simulink model "TCS_autosar"  (R2019b)
settings: Solver=VariableStepAuto  StartTime=0.0  StopTime=10.0  RelTol=1e-3
libraries: simulink x20
settings Model: Creator=12045  LastModifiedBy=12045
settings OptimizationCC: DefaultParameterBehavior=Inlined  EnhancedBackFolding=on  PassReuseOutputArgsAs=Individual arguments  ZeroExternalMemoryAtStartup=off  ZeroInternalMemoryAtStartup=off  OptimizeBlockOrder=speed  DifferentSizesBufferReuse=on  OptimizationCustomize=off  EfficientTunableParamExpr=on
settings DebuggingCC: ParameterTunabilityLossMsg=error
settings SFSimCC: SimGenImportedTypeDefs=on  MATLABDynamicMemAlloc=off
settings RTWCC: Description=AUTOSAR  SystemTargetFile=autosar.tlc  GenCodeOnly=on  TemplateMakefile=ert_default_tmf  GenerateReport=on  Toolchain=AUTOSAR Adaptive | CMake  IncludeHyperlinkInReport=on  LaunchReport=on  GenerateTraceInfo=on  GenerateTraceReport=on  GenerateTraceReportSl=on  GenerateTraceReportSf=on  GenerateTraceReportEml=on
settings CodeAppCC: ForceParamTrailComments=on  IgnoreCustomStorageClasses=off  MaxIdLength=63  OperatorAnnotations=on  SimulinkDataObjDesc=on  SFDataObjDesc=on  InsertBlockDesc=on
settings STFCustomTargetCC: TargetLangStandard=C99 (ISO)  MultiwordLength=256  ParMdlRefBuildCompliant=on  CompOptLevelCompliant=on  IncludeMdlTerminateFcn=off  CombineOutputUpdateFcns=on  SuppressErrorStatus=on  ERTCustomFileBanners=on  SupportNonFinite=off  SupportComplex=off  SupportContinuousTime=off  SupportNonInlinedSFcns=off  RemoveResetFunc=on  MATLABClassNameForMDSCustomization=Simulink.SoftwareTarget.ERTCustomization  AutosarCompliant=on  UseToolchainInfoCompliant=on  LookupTableObjectStructAxisOrder=2,1,3,4,...  LUTObjectStructOrderEvenSpacing=Size,Table,Breakpoints  SystemTargetFile=autosar.tlc
settings ERTTargetCC: TargetLangStandard=C99 (ISO)  ConcurrentExecutionCompliant=off  IncludeMdlTerminateFcn=off  SuppressErrorStatus=on  SupportNonFinite=off  SupportComplex=off  ModelStepFunctionPrototypeControlCompliant=off  CPPClassGenCompliant=off  AutosarCompliant=on  LookupTableObjectStructAxisOrder=2,1,3,4,...  LUTObjectStructOrderEvenSpacing=Size,Table,Breakpoints  InlinedParameterPlacement=NonHierarchical  ERTCustomFileTemplate=example_file_process.tlc

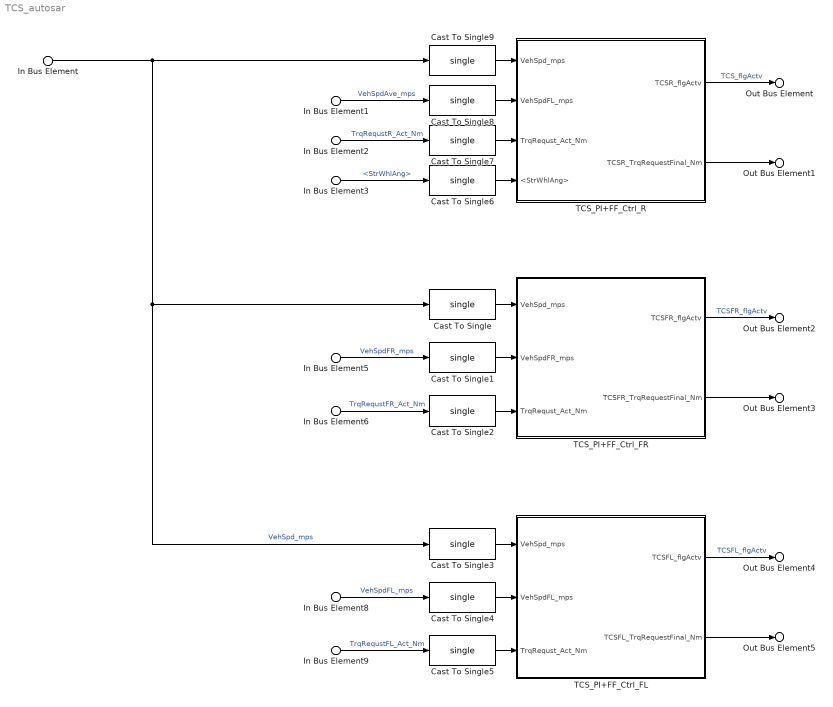
== system TCS_autosar ==
  In Bus Element : Inport  PortName=VehSpd_mps  Element=VehSpd_mps
  In Bus Element1 : Inport  Port=2  PortName=VehSpdAve_mps  Element=VehSpdAve_mps
  In Bus Element2 : Inport  Port=3  PortName=TrqRequstR_Act_Nm  Element=TrqRequstR_Act_Nm
  In Bus Element3 : Inport  Port=4  PortName=StrWhlAng  Element=StrWhlAng
  In Bus Element5 : Inport  Port=5  PortName=VehSpdFR_mps  Element=VehSpdFR_mps
  In Bus Element6 : Inport  Port=6  PortName=TrqRequstFR_Act_Nm  Element=TrqRequstFR_Act_Nm
  In Bus Element8 : Inport  Port=7  PortName=VehSpdFL_mps1  Element=VehSpdFL_mpsVehSpdFL_mps1
  In Bus Element9 : Inport  Port=8  PortName=TrqRequst_Act_Nm2  Element=TrqRequstFL_Act_NmTrqRequstFL_Act_Nm
  Cast To Single{,1..9} (10 alike) : DataTypeConversion  OutDataTypeStr=single
  TCS_PI+FF_Ctrl_FL : Subsystem
  TCS_PI+FF_Ctrl_FR : Subsystem
  TCS_PI+FF_Ctrl_R : Subsystem
  Out Bus Element : Outport  PortName=TCS_flgActv_R  Element=TCS_flgActv_R
  Out Bus Element1 : Outport  Port=2  PortName=TCSR_TrqRequestFinal_Nm  Element=TCSR_TrqRequestFinal_Nm
  Out Bus Element2 : Outport  Port=3  PortName=TCS_flgActv_FR  Element=TCS_flgActv_FR
  Out Bus Element3 : Outport  Port=4  PortName=TCSFR_TrqRequestFinal_Nm  Element=TCSFR_TrqRequestFinal_Nm
  Out Bus Element4 : Outport  Port=5  PortName=TCS_flgActv_FL  Element=TCS_flgActv_FL
  Out Bus Element5 : Outport  Port=6  PortName=TCSFL_TrqRequestFinal_Nm  Element=TCSFL_TrqRequestFinal_Nm
  wires:
  Cast To Single/1 -> TCS_PI+FF_Ctrl_FR/1(VehSpd_mps)
  Cast To Single1/1 -> TCS_PI+FF_Ctrl_FR/2(VehSpdFR_mps)
  Cast To Single2/1 -> TCS_PI+FF_Ctrl_FR/3(TrqRequst_Act_Nm)
  Cast To Single3/1 -> TCS_PI+FF_Ctrl_FL/1(VehSpd_mps)
  Cast To Single4/1 -> TCS_PI+FF_Ctrl_FL/2(VehSpdFL_mps)
  Cast To Single5/1 -> TCS_PI+FF_Ctrl_FL/3(TrqRequst_Act_Nm)
  Cast To Single6/1 -> TCS_PI+FF_Ctrl_R/4(<StrWhlAng>)
  Cast To Single7/1 -> TCS_PI+FF_Ctrl_R/3(TrqRequst_Act_Nm)
  Cast To Single8/1 -> TCS_PI+FF_Ctrl_R/2(VehSpdFL_mps)
  Cast To Single9/1 -> TCS_PI+FF_Ctrl_R/1(VehSpd_mps)
  In Bus Element/1 -> Cast To Single3/1, Cast To Single/1, Cast To Single9/1  "VehSpd_mps"
  In Bus Element1/1 -> Cast To Single8/1  "VehSpdAve_mps"
  In Bus Element2/1 -> Cast To Single7/1  "TrqRequstR_Act_Nm"
  In Bus Element3/1 -> Cast To Single6/1  "<StrWhlAng>"
  In Bus Element5/1 -> Cast To Single1/1  "VehSpdFR_mps"
  In Bus Element6/1 -> Cast To Single2/1  "TrqRequstFR_Act_Nm"
  In Bus Element8/1 -> Cast To Single4/1  "VehSpdFL_mps"
  In Bus Element9/1 -> Cast To Single5/1  "TrqRequstFL_Act_Nm"
  TCS_PI+FF_Ctrl_R/1(TCSR_flgActv) -> Out Bus Element/1  "TCS_flgActv"
  TCS_PI+FF_Ctrl_R/2(TCSR_TrqRequestFinal_Nm) -> Out Bus Element1/1
  TCS_PI+FF_Ctrl_FR/1(TCSFR_flgActv) -> Out Bus Element2/1  "TCSFR_flgActv"
  TCS_PI+FF_Ctrl_FR/2(TCSFR_TrqRequestFinal_Nm) -> Out Bus Element3/1
  TCS_PI+FF_Ctrl_FL/1(TCSFL_flgActv) -> Out Bus Element4/1  "TCSFL_flgActv"
  TCS_PI+FF_Ctrl_FL/2(TCSFL_TrqRequestFinal_Nm) -> Out Bus Element5/1

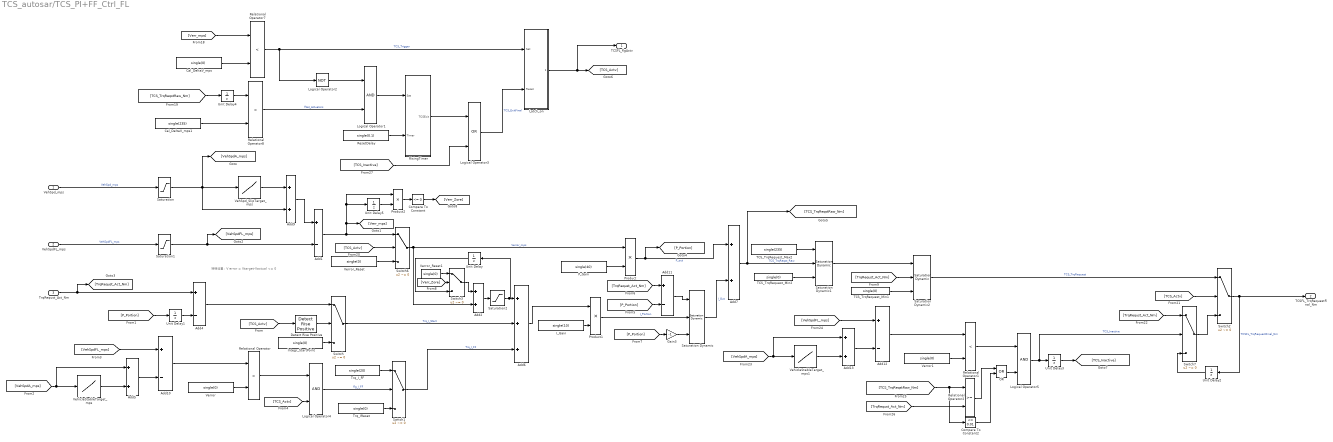
== system TCS_autosar/TCS_PI+FF_Ctrl_FL ==
  note: 特殊设置：V error = Vtarget-Vactual <= 0
  VehSpd_mps : Inport
  VehSpdFL_mps : Inport  Port=2
  TrqRequst_Act_Nm : Inport  Port=3
  Add{1,4,10..12} (5 alike) : Sum  Inputs=+-
  Add{2,5,7,9,13} (5 alike) : Sum
  Add6 : Sum  Inputs=+++
  Cal_DeltaV_mps : Constant  Value=single(0)
  Cal_DeltaV_mps1 : Constant  Value=single(235)
  Compare To Constant : simulink/Logic and Bit Operations/Compare To Constant  relop=<=  const=0  OutDataTypeStr=boolean
  Compare To Constant2 : simulink/Logic and Bit Operations/Compare To Constant  relop=<=  const=0.01  OutDataTypeStr=boolean
  Detect Rise Positive : simulink/Logic and Bit Operations/Detect Rise Positive  vinit=0  OutDataTypeStr=boolean
  Gain3 : Gain  Gain=-1
  I_Gain : Constant  Value=single(10)
  Integr_StartPoint : Constant  Value=single(0)
  Latch_on : Subsystem
  Logical Operator1 : Logic  AllPortsSameDT=off  OutDataTypeStr=boolean
  Logical Operator2 : Logic  Operator=NOT  AllPortsSameDT=off  OutDataTypeStr=boolean
  Logical Operator3 : Logic  Operator=OR  AllPortsSameDT=off  OutDataTypeStr=boolean
  Logical Operator4 : Logic  AllPortsSameDT=off  OutDataTypeStr=boolean
  Logical Operator5 : Logic  AllPortsSameDT=off  OutDataTypeStr=boolean
  OR : Logic  Operator=OR  AllPortsSameDT=off  OutDataTypeStr=boolean
  P_Gain : Constant  Value=single(40)
  Product : Product
  Product1 : Product
  Product2 : Product
  Relational Operator : RelationalOperator  Operator=<  OutDataTypeStr=boolean  RndMeth=Simplest
  Relational Operator1 : RelationalOperator  Operator=<  OutDataTypeStr=boolean  RndMeth=Simplest
  Relational Operator2 : RelationalOperator  OutDataTypeStr=boolean  RndMeth=Simplest
  Relational Operator7 : RelationalOperator  Operator=<  OutDataTypeStr=boolean  RndMeth=Simplest
  Relational Operator8 : RelationalOperator  Operator=>  OutDataTypeStr=boolean  RndMeth=Simplest
  ResetDelay : Constant  Value=single(0.1)
  RisingTimer : Subsystem
  Saturation : Saturate  UpperLimit=40  LowerLimit=0
  Saturation Dynamic : simulink/Discontinuities/Saturation Dynamic  OutMin=[]  OutMax=[]  OutDataTypeStr=Inherit: Same as second input  OutDataType=fixdt(1, 16)  OutScaling=2^-10  DoSatur=off
  Saturation Dynamic1 : simulink/Discontinuities/Saturation Dynamic  OutMin=[]  OutMax=[]  OutDataTypeStr=Inherit: Same as second input  OutDataType=fixdt(1, 16)  OutScaling=2^-10  DoSatur=off
  Saturation Dynamic2 : simulink/Discontinuities/Saturation Dynamic  OutMin=[]  OutMax=[]  OutDataTypeStr=Inherit: Same as second input  OutDataType=fixdt(1, 16)  OutScaling=2^-10  DoSatur=off
  Saturation1 : Saturate  UpperLimit=50  LowerLimit=0
  Saturation2 : Saturate  UpperLimit=400  LowerLimit=-100
  Switch{,1..3,6..7} (6 alike) : Switch  Criteria=u2 ~= 0
  TCS_TrqRequest_Max2 : Constant  Value=single(235)
  TCS_TrqRequest_Min1 : Constant  Value=single(0)
  TCS_TrqRequest_Min2 : Constant  Value=single(0)
  Trq_IReset : Constant  Value=single(0)
  Trq_I_FF : Constant  Value=single(20)
  Unit Delay{,1..5} (6 alike) : UnitDelay  SampleTime=-1  HasFrameUpgradeWarning=on
  VehSpd_SlipTarget_mps : Lookup_n-D  NumberOfTableDimensions=1  BreakpointsForDimension1=[0,3,25,30]  Table=[0.3,0.3,2.5,2.5]  ExtrapMethod=Clip  InternalRulePriority=Speed  RndMeth=Simplest  InputSameDT=on
  VehicleStableTarget_mps : Lookup_n-D  NumberOfTableDimensions=1  BreakpointsForDimension1=[0,3,25,30]  Table=[0.4,0.4,1.2,1.2]  ExtrapMethod=Clip  InternalRulePriority=Speed  RndMeth=Simplest  InputSameDT=on
  VehicleStableTarget_mps1 : Lookup_n-D  NumberOfTableDimensions=1  BreakpointsForDimension1=[0,3,25,30]  Table=[0.4,0.4,1.2,1.2]  ExtrapMethod=Clip  InternalRulePriority=Speed  RndMeth=Simplest  InputSameDT=on
  Verror : Constant  Value=single(0)
  Verror1 : Constant  Value=single(0)
  Verror_Reset : Constant  Value=single(0)
  Verror_Reset1 : Constant  Value=single(0)
  TCSFL_flgActv : Outport
  TCSFL_TrqRequestFinal_Nm : Outport  Port=2
  wires:
  Switch2/1 -> TCSFL_TrqRequestFinal_Nm/1, Unit Delay2/1  "TCSFL_TrqRequestFinal_Nm"
  Saturation/1 -> Add9/2, VehSpd_SlipTarget_mps/1, [VehSpdA_mps]
  Gain3/1 -> Saturation Dynamic/3
  [P_Portion] -> Gain3/1
  P_Gain/1 -> Product/2
  Unit Delay/1 -> Switch3/3
  Add2/1 -> Saturation2/1
  [TrqRequst_Act_Nm] -> Add11/1
  Saturation2/1 -> Unit Delay/1, Add6/1
  Switch/1 -> Add6/2  "Trq_I_Start"
  Saturation Dynamic/1 -> Add7/2  "I_Out"
  VehSpd_mps/1 -> Saturation/1  "VehSpd_mps"
  Saturation1/1 -> Add1/2, [VehSpdFL_mps]
  Product1/1 -> Saturation Dynamic/2  "I_Portion"
  TrqRequst_Act_Nm/1 -> Add4/1, [TrqRequst_Act_Nm]
  Add6/1 -> Product1/1
  TCS_TrqRequest_Min1/1 -> Saturation Dynamic2/3
  Detect Rise Positive/1 -> Switch/2
  Integr_StartPoint/1 -> Switch/3
  I_Gain/1 -> Product1/2
  Saturation Dynamic2/1 -> Switch2/1  "TCS_TrqRequest"
  Add7/1 -> Saturation Dynamic1/2, [TCS_TrqReqstRaw_Nm]  "TCS_TrqReqst_Raw"
  [TrqRequst_Act_Nm] -> Saturation Dynamic2/2
  VehSpd_SlipTarget_mps/1 -> Add9/1
  Add9/1 -> Add1/1
  [Verr_mps] -> Relational Operator7/1
  Cal_DeltaV_mps/1 -> Relational Operator7/2
  Relational Operator7/1 -> Latch_on/1(Set), Logical Operator2/1  "TCS_Trigger"
  [TCS_TrqReqstRaw_Nm] -> Unit Delay4/1
  Logical Operator2/1 -> Logical Operator1/1
  Relational Operator8/1 -> Logical Operator1/2  "fSat_Actuators"
  Cal_DeltaV_mps1/1 -> Relational Operator8/2
  Logical Operator1/1 -> RisingTimer/1(Set)
  ResetDelay/1 -> RisingTimer/2(Timer)
  RisingTimer/1(TCSExit) -> Logical Operator3/1
  Logical Operator3/1 -> Latch_on/2(Reset)  "TCS_ExitFinal"
  Latch_on/1(flg_TCSActv) -> TCSFL_flgActv/1, [TCS_Actv]
  [TCS_Actv] -> Switch6/2
  Verror_Reset/1 -> Switch6/3
  Switch6/1 -> Product/1, Add2/2  "Verror_mps"
  Product/1 -> [P_Portion], Add7/1  "P_out"
  [TCS_Actv] -> Detect Rise Positive/1
  [P_Portion] -> Unit Delay1/1
  Add4/1 -> Switch/1
  Unit Delay1/1 -> Add4/2
  [VehSpdA_mps] -> Add5/1, VehicleStableTarget_mps/1
  VehicleStableTarget_mps/1 -> Add5/2
  Add5/1 -> Add10/2
  [VehSpdFL_mps] -> Add10/1
  Add10/1 -> Relational Operator/1
  Verror/1 -> Relational Operator/2
  Relational Operator/1 -> Logical Operator4/1
  [TCS_Actv] -> Logical Operator4/2
  Logical Operator4/1 -> Switch1/2  "flg_I_FF"
  Trq_I_FF/1 -> Switch1/1
  Trq_IReset/1 -> Switch1/3
  Switch1/1 -> Add6/3  "Trq_I_FF"
  [P_Portion] -> Add11/2
  Add11/1 -> Saturation Dynamic/1
  [TCS_Actv] -> Switch2/2
  Switch7/1 -> Switch2/3
  [TrqRequst_Act_Nm] -> Switch7/1
  Verror1/1 -> Relational Operator1/2
  Add12/1 -> Relational Operator1/1
  [VehSpdFL_mps] -> Add12/1
  Add13/1 -> Add12/2
  VehicleStableTarget_mps1/1 -> Add13/2
  [VehSpdA_mps] -> VehicleStableTarget_mps1/1, Add13/1
  [TCS_TrqReqstRaw_Nm] -> Compare To Constant2/1, Relational Operator2/1
  [TrqRequst_Act_Nm] -> Relational Operator2/2
  Relational Operator1/1 -> Logical Operator5/1
  Logical Operator5/1 -> Switch7/2, Unit Delay3/1  "TCS_Inactive"
  Unit Delay3/1 -> [TCS_Inactive]
  [TCS_Inactive] -> Logical Operator3/2
  Unit Delay4/1 -> Relational Operator8/1
  VehSpdFL_mps/1 -> Saturation1/1  "VehSpdFL_mps"
  Saturation Dynamic1/1 -> Saturation Dynamic2/1
  TCS_TrqRequest_Max2/1 -> Saturation Dynamic1/1
  TCS_TrqRequest_Min2/1 -> Saturation Dynamic1/3
  Switch3/1 -> Add2/1
  Verror_Reset1/1 -> Switch3/1
  [Verr_Zore] -> Switch3/2
  Product2/1 -> Compare To Constant/1
  Unit Delay5/1 -> Product2/2
  Add1/1 -> Switch6/1, [Verr_mps], Unit Delay5/1, Product2/1
  Compare To Constant/1 -> [Verr_Zore]
  Unit Delay2/1 -> Switch7/3
  Compare To Constant2/1 -> OR/2
  Relational Operator2/1 -> OR/1
  OR/1 -> Logical Operator5/2

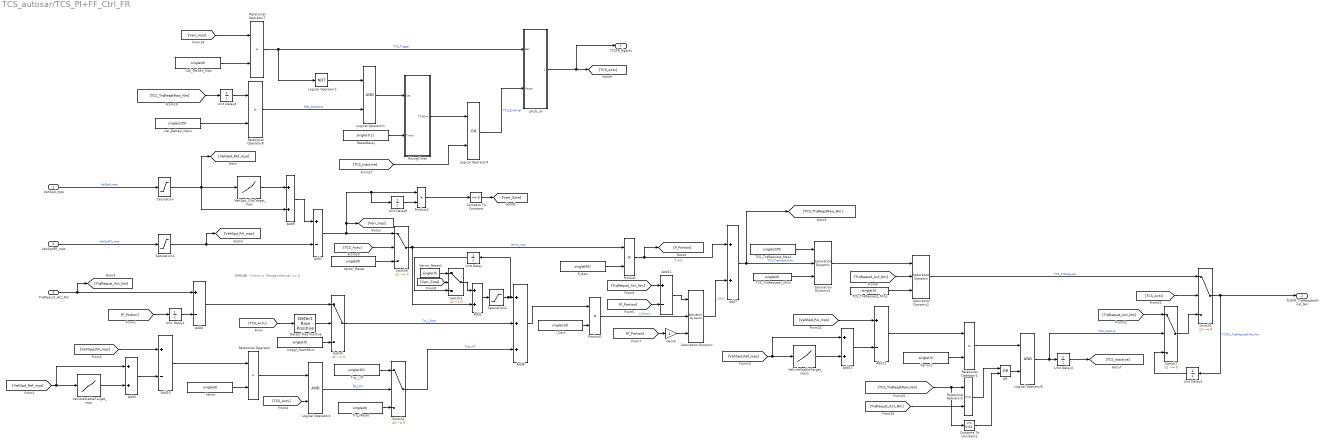
== system TCS_autosar/TCS_PI+FF_Ctrl_FR ==
  note: 特殊设置：V error = Vtarget-Vactual <= 0
  VehSpd_mps : Inport
  VehSpdFR_mps : Inport  Port=2
  TrqRequst_Act_Nm : Inport  Port=3
  Add{1,4,10..12} (5 alike) : Sum  Inputs=+-
  Add{2,5,7,9,13} (5 alike) : Sum
  Add6 : Sum  Inputs=+++
  Cal_DeltaV_mps : Constant  Value=single(0)
  Cal_DeltaV_mps1 : Constant  Value=single(235)
  Compare To Constant : simulink/Logic and Bit Operations/Compare To Constant  relop=<=  const=0  OutDataTypeStr=boolean
  Compare To Constant2 : simulink/Logic and Bit Operations/Compare To Constant  relop=<=  const=0.01  OutDataTypeStr=boolean
  Detect Rise Positive : simulink/Logic and Bit Operations/Detect Rise Positive  vinit=0  OutDataTypeStr=boolean
  Gain3 : Gain  Gain=-1
  I_Gain : Constant  Value=single(10)
  Integr_StartPoint : Constant  Value=single(0)
  Latch_on : Subsystem
  Logical Operator1 : Logic  AllPortsSameDT=off  OutDataTypeStr=boolean
  Logical Operator2 : Logic  Operator=NOT  AllPortsSameDT=off  OutDataTypeStr=boolean
  Logical Operator3 : Logic  Operator=OR  AllPortsSameDT=off  OutDataTypeStr=boolean
  Logical Operator4 : Logic  AllPortsSameDT=off  OutDataTypeStr=boolean
  Logical Operator5 : Logic  AllPortsSameDT=off  OutDataTypeStr=boolean
  OR : Logic  Operator=OR  AllPortsSameDT=off  OutDataTypeStr=boolean
  P_Gain : Constant  Value=single(40)
  Product : Product
  Product1 : Product
  Product2 : Product
  Relational Operator : RelationalOperator  Operator=<  OutDataTypeStr=boolean  RndMeth=Simplest
  Relational Operator1 : RelationalOperator  Operator=<  OutDataTypeStr=boolean  RndMeth=Simplest
  Relational Operator2 : RelationalOperator  OutDataTypeStr=boolean  RndMeth=Simplest
  Relational Operator7 : RelationalOperator  Operator=<  OutDataTypeStr=boolean  RndMeth=Simplest
  Relational Operator8 : RelationalOperator  Operator=>  OutDataTypeStr=boolean  RndMeth=Simplest
  ResetDelay : Constant  Value=single(0.1)
  RisingTimer : Subsystem
  Saturation : Saturate  UpperLimit=40  LowerLimit=0
  Saturation Dynamic : simulink/Discontinuities/Saturation Dynamic  OutMin=[]  OutMax=[]  OutDataTypeStr=Inherit: Same as second input  OutDataType=fixdt(1, 16)  OutScaling=2^-10  DoSatur=off
  Saturation Dynamic1 : simulink/Discontinuities/Saturation Dynamic  OutMin=[]  OutMax=[]  OutDataTypeStr=Inherit: Same as second input  OutDataType=fixdt(1, 16)  OutScaling=2^-10  DoSatur=off
  Saturation Dynamic2 : simulink/Discontinuities/Saturation Dynamic  OutMin=[]  OutMax=[]  OutDataTypeStr=Inherit: Same as second input  OutDataType=fixdt(1, 16)  OutScaling=2^-10  DoSatur=off
  Saturation1 : Saturate  UpperLimit=50  LowerLimit=0
  Saturation2 : Saturate  UpperLimit=400  LowerLimit=-100
  Switch{,1..3,6..7} (6 alike) : Switch  Criteria=u2 ~= 0
  TCS_TrqRequest_Max2 : Constant  Value=single(235)
  TCS_TrqRequest_Min1 : Constant  Value=single(0)
  TCS_TrqRequest_Min2 : Constant  Value=single(0)
  Trq_IReset : Constant  Value=single(0)
  Trq_I_FF : Constant  Value=single(20)
  Unit Delay{,1..5} (6 alike) : UnitDelay  SampleTime=-1  HasFrameUpgradeWarning=on
  VehSpd_SlipTarget_mps : Lookup_n-D  NumberOfTableDimensions=1  BreakpointsForDimension1=[0,3,25,30]  Table=[0.3,0.3,2.5,2.5]  ExtrapMethod=Clip  InternalRulePriority=Speed  RndMeth=Simplest  InputSameDT=on
  VehicleStableTarget_mps : Lookup_n-D  NumberOfTableDimensions=1  BreakpointsForDimension1=[0,3,25,30]  Table=[0.4,0.4,1.2,1.2]  ExtrapMethod=Clip  InternalRulePriority=Speed  RndMeth=Simplest  InputSameDT=on
  VehicleStableTarget_mps1 : Lookup_n-D  NumberOfTableDimensions=1  BreakpointsForDimension1=[0,3,25,30]  Table=[0.4,0.4,1.2,1.2]  ExtrapMethod=Clip  InternalRulePriority=Speed  RndMeth=Simplest  InputSameDT=on
  Verror : Constant  Value=single(0)
  Verror1 : Constant  Value=single(0)
  Verror_Reset : Constant  Value=single(0)
  Verror_Reset1 : Constant  Value=single(0)
  TCSFR_flgActv : Outport
  TCSFR_TrqRequestFinal_Nm : Outport  Port=2
  wires:
  [Verr_Zore] -> Switch3/2
  Verror_Reset1/1 -> Switch3/1
  Switch3/1 -> Add2/1
  TCS_TrqRequest_Min2/1 -> Saturation Dynamic1/3
  TCS_TrqRequest_Max2/1 -> Saturation Dynamic1/1
  Saturation Dynamic1/1 -> Saturation Dynamic2/1
  VehSpdFR_mps/1 -> Saturation1/1  "VehSpdFL_mps"
  Unit Delay4/1 -> Relational Operator8/1
  [TCS_Inactive] -> Logical Operator3/2
  Unit Delay3/1 -> [TCS_Inactive]
  Logical Operator5/1 -> Switch7/2, Unit Delay3/1  "TCS_Inactive"
  Relational Operator1/1 -> Logical Operator5/1
  [TrqRequst_Act_Nm] -> Relational Operator2/2
  [TCS_TrqReqstRaw_Nm] -> Compare To Constant2/1, Relational Operator2/1
  [VehSpd_Ref_mps] -> Add13/1, VehicleStableTarget_mps1/1
  VehicleStableTarget_mps1/1 -> Add13/2
  Add13/1 -> Add12/2
  [VehSpd_RA_mps] -> Add12/1
  Add12/1 -> Relational Operator1/1
  Verror1/1 -> Relational Operator1/2
  [TrqRequst_Act_Nm] -> Switch7/1
  Switch7/1 -> Switch2/3
  [TCS_Actv] -> Switch2/2
  Add11/1 -> Saturation Dynamic/1
  [P_Portion] -> Add11/2
  Switch1/1 -> Add6/3  "Trq_I_FF"
  Trq_IReset/1 -> Switch1/3
  Trq_I_FF/1 -> Switch1/1
  Logical Operator4/1 -> Switch1/2  "flg_I_FF"
  [TCS_Actv] -> Logical Operator4/2
  Relational Operator/1 -> Logical Operator4/1
  Verror/1 -> Relational Operator/2
  Add10/1 -> Relational Operator/1
  [VehSpd_RA_mps] -> Add10/1
  Add5/1 -> Add10/2
  VehicleStableTarget_mps/1 -> Add5/2
  [VehSpd_Ref_mps] -> VehicleStableTarget_mps/1, Add5/1
  Unit Delay1/1 -> Add4/2
  Add4/1 -> Switch/1
  [P_Portion] -> Unit Delay1/1
  [TCS_Actv] -> Detect Rise Positive/1
  Product/1 -> Add7/1, [P_Portion]  "P_out"
  Switch6/1 -> Add2/2, Product/1  "Verror_mps"
  Verror_Reset/1 -> Switch6/3
  [TCS_Actv] -> Switch6/2
  Latch_on/1(flg_TCSActv) -> [TCS_Actv], TCSFR_flgActv/1
  Logical Operator3/1 -> Latch_on/2(Reset)  "TCS_ExitFinal"
  RisingTimer/1(TCSExit) -> Logical Operator3/1
  ResetDelay/1 -> RisingTimer/2(Timer)
  Logical Operator1/1 -> RisingTimer/1(Set)
  Cal_DeltaV_mps1/1 -> Relational Operator8/2
  Relational Operator8/1 -> Logical Operator1/2  "fSat_Actuators"
  Logical Operator2/1 -> Logical Operator1/1
  [TCS_TrqReqstRaw_Nm] -> Unit Delay4/1
  Relational Operator7/1 -> Logical Operator2/1, Latch_on/1(Set)  "TCS_Trigger"
  Cal_DeltaV_mps/1 -> Relational Operator7/2
  [Verr_mps] -> Relational Operator7/1
  Add9/1 -> Add1/1
  VehSpd_SlipTarget_mps/1 -> Add9/1
  [TrqRequst_Act_Nm] -> Saturation Dynamic2/2
  Add7/1 -> [TCS_TrqReqstRaw_Nm], Saturation Dynamic1/2  "TCS_TrqReqst_Raw"
  Saturation Dynamic2/1 -> Switch2/1  "TCS_TrqRequest"
  I_Gain/1 -> Product1/2
  Integr_StartPoint/1 -> Switch/3
  Detect Rise Positive/1 -> Switch/2
  TCS_TrqRequest_Min1/1 -> Saturation Dynamic2/3
  Add6/1 -> Product1/1
  TrqRequst_Act_Nm/1 -> [TrqRequst_Act_Nm], Add4/1
  Product1/1 -> Saturation Dynamic/2  "I_Portion"
  Saturation1/1 -> [VehSpd_RA_mps], Add1/2
  VehSpd_mps/1 -> Saturation/1  "VehSpd_mps"
  Saturation Dynamic/1 -> Add7/2  "I_Out"
  Switch/1 -> Add6/2  "Trq_I_Start"
  Saturation2/1 -> Add6/1, Unit Delay/1
  [TrqRequst_Act_Nm] -> Add11/1
  Add2/1 -> Saturation2/1
  Unit Delay/1 -> Switch3/3
  P_Gain/1 -> Product/2
  [P_Portion] -> Gain3/1
  Gain3/1 -> Saturation Dynamic/3
  Saturation/1 -> [VehSpd_Ref_mps], VehSpd_SlipTarget_mps/1, Add9/2
  Switch2/1 -> Unit Delay2/1, TCSFR_TrqRequestFinal_Nm/1  "TCSFL_TrqRequestFinal_Nm"
  Product2/1 -> Compare To Constant/1
  Unit Delay5/1 -> Product2/2
  Add1/1 -> Unit Delay5/1, Product2/1, [Verr_mps], Switch6/1
  Compare To Constant/1 -> [Verr_Zore]
  Unit Delay2/1 -> Switch7/3
  Compare To Constant2/1 -> OR/2
  Relational Operator2/1 -> OR/1
  OR/1 -> Logical Operator5/2

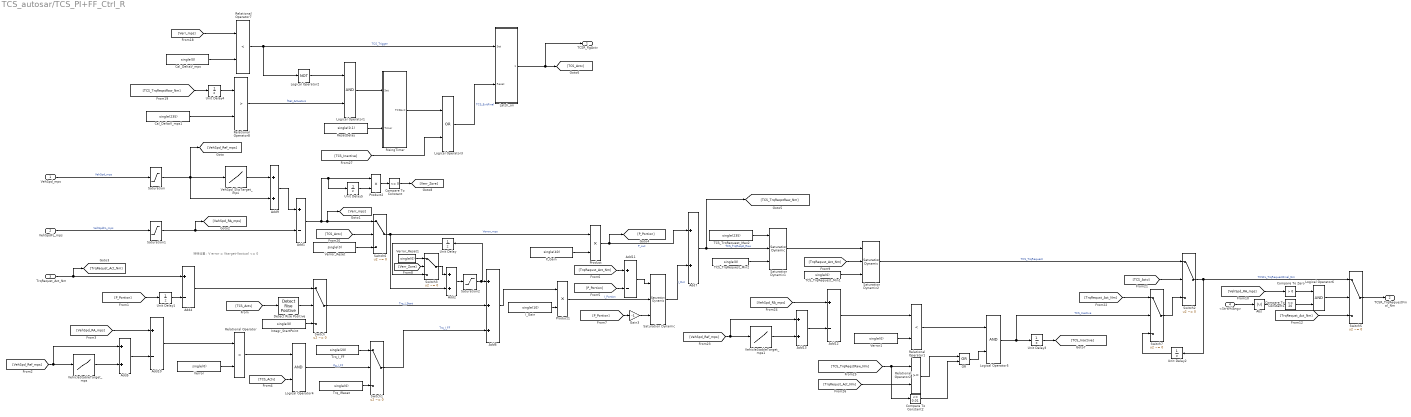
== system TCS_autosar/TCS_PI+FF_Ctrl_R ==
  note: 特殊设置：V error = Vtarget-Vactual <= 0
  VehSpd_mps : Inport
  VehSpdFL_mps : Inport  Port=2
  TrqRequst_Act_Nm : Inport  Port=3
  <StrWhlAng> : Inport  Port=4
  Abs : Abs
  Add{1,4,10..12} (5 alike) : Sum  Inputs=+-
  Add{2,5,7,9,13} (5 alike) : Sum
  Add6 : Sum  Inputs=+++
  Cal_DeltaV_mps : Constant  Value=single(0)
  Cal_DeltaV_mps1 : Constant  Value=single(235)
  Compare To Constant : simulink/Logic and Bit Operations/Compare To Constant  relop=<=  const=0  OutDataTypeStr=boolean
  Compare To Constant1 : simulink/Logic and Bit Operations/Compare To Constant  relop=<=  const=20  OutDataTypeStr=boolean
  Compare To Constant2 : simulink/Logic and Bit Operations/Compare To Constant  relop=<=  const=0.01  OutDataTypeStr=boolean
  Compare To Zero : simulink/Logic and Bit Operations/Compare To Zero  relop=>  OutDataTypeStr=boolean
  Detect Rise Positive : simulink/Logic and Bit Operations/Detect Rise Positive  vinit=0  OutDataTypeStr=boolean
  Gain3 : Gain  Gain=-1
  I_Gain : Constant  Value=single(10)
  Integr_StartPoint : Constant  Value=single(0)
  Latch_on : Subsystem
  Logical Operator{1,4..6} (4 alike) : Logic  AllPortsSameDT=off  OutDataTypeStr=boolean
  Logical Operator2 : Logic  Operator=NOT  AllPortsSameDT=off  OutDataTypeStr=boolean
  Logical Operator3 : Logic  Operator=OR  AllPortsSameDT=off  OutDataTypeStr=boolean
  OR : Logic  Operator=OR  AllPortsSameDT=off  OutDataTypeStr=boolean
  P_Gain : Constant  Value=single(40)
  Product : Product
  Product1 : Product
  Product2 : Product
  Relational Operator : RelationalOperator  Operator=<  OutDataTypeStr=boolean  RndMeth=Simplest
  Relational Operator1 : RelationalOperator  Operator=<  OutDataTypeStr=boolean  RndMeth=Simplest
  Relational Operator2 : RelationalOperator  OutDataTypeStr=boolean  RndMeth=Simplest
  Relational Operator7 : RelationalOperator  Operator=<  OutDataTypeStr=boolean  RndMeth=Simplest
  Relational Operator8 : RelationalOperator  Operator=>  OutDataTypeStr=boolean  RndMeth=Simplest
  ResetDelay : Constant  Value=single(0.1)
  RisingTimer : Subsystem
  Saturation : Saturate  UpperLimit=40  LowerLimit=0
  Saturation Dynamic : simulink/Discontinuities/Saturation Dynamic  OutMin=[]  OutMax=[]  OutDataTypeStr=Inherit: Same as second input  OutDataType=fixdt(1, 16)  OutScaling=2^-10  DoSatur=off
  Saturation Dynamic1 : simulink/Discontinuities/Saturation Dynamic  OutMin=[]  OutMax=[]  OutDataTypeStr=Inherit: Same as second input  OutDataType=fixdt(1, 16)  OutScaling=2^-10  DoSatur=off
  Saturation Dynamic2 : simulink/Discontinuities/Saturation Dynamic  OutMin=[]  OutMax=[]  OutDataTypeStr=Inherit: Same as second input  OutDataType=fixdt(1, 16)  OutScaling=2^-10  DoSatur=off
  Saturation1 : Saturate  UpperLimit=50  LowerLimit=0
  Saturation2 : Saturate  UpperLimit=400  LowerLimit=-100
  Switch{,1..3,5..7} (7 alike) : Switch  Criteria=u2 ~= 0
  TCS_TrqRequest_Max2 : Constant  Value=single(235)
  TCS_TrqRequest_Min1 : Constant  Value=single(0)
  TCS_TrqRequest_Min2 : Constant  Value=single(0)
  Trq_IReset : Constant  Value=single(0)
  Trq_I_FF : Constant  Value=single(20)
  Unit Delay{,1..5} (6 alike) : UnitDelay  SampleTime=-1  HasFrameUpgradeWarning=on
  VehSpd_SlipTarget_mps : Lookup_n-D  NumberOfTableDimensions=1  BreakpointsForDimension1=[0,3,25,30]  Table=[0.3,0.3,2.5,2.5]  ExtrapMethod=Clip  InternalRulePriority=Speed  RndMeth=Simplest  InputSameDT=on
  VehicleStableTarget_mps : Lookup_n-D  NumberOfTableDimensions=1  BreakpointsForDimension1=[0,3,25,30]  Table=[0.4,0.4,1.2,1.2]  ExtrapMethod=Clip  InternalRulePriority=Speed  RndMeth=Simplest  InputSameDT=on
  VehicleStableTarget_mps1 : Lookup_n-D  NumberOfTableDimensions=1  BreakpointsForDimension1=[0,3,25,30]  Table=[0.4,0.4,1.2,1.2]  ExtrapMethod=Clip  InternalRulePriority=Speed  RndMeth=Simplest  InputSameDT=on
  Verror : Constant  Value=single(0)
  Verror1 : Constant  Value=single(0)
  Verror_Reset : Constant  Value=single(0)
  Verror_Reset1 : Constant  Value=single(0)
  TCSR_flgActv : Outport
  TCSR_TrqRequestFinal_Nm : Outport  Port=2
  wires:
  Add1/1 -> Unit Delay5/1, Product2/1, Switch6/1, [Verr_mps]
  Switch2/1 -> Switch5/1, Unit Delay2/1  "TCSFL_TrqRequestFinal_Nm"
  Saturation/1 -> Add9/2, VehSpd_SlipTarget_mps/1, [VehSpd_Ref_mps]
  Gain3/1 -> Saturation Dynamic/3
  [P_Portion] -> Gain3/1
  P_Gain/1 -> Product/2
  Unit Delay/1 -> Switch3/3
  Add2/1 -> Saturation2/1
  [TrqRequst_Act_Nm] -> Add11/1
  Saturation2/1 -> Unit Delay/1, Add6/1
  Switch/1 -> Add6/2  "Trq_I_Start"
  Saturation Dynamic/1 -> Add7/2  "I_Out"
  VehSpd_mps/1 -> Saturation/1  "VehSpd_mps"
  Saturation1/1 -> Add1/2, [VehSpd_RA_mps]
  Product1/1 -> Saturation Dynamic/2  "I_Portion"
  TrqRequst_Act_Nm/1 -> Add4/1, [TrqRequst_Act_Nm]
  Add6/1 -> Product1/1
  TCS_TrqRequest_Min1/1 -> Saturation Dynamic2/3
  Detect Rise Positive/1 -> Switch/2
  Integr_StartPoint/1 -> Switch/3
  I_Gain/1 -> Product1/2
  Saturation Dynamic2/1 -> Switch2/1  "TCS_TrqRequest"
  Add7/1 -> Saturation Dynamic1/2, [TCS_TrqReqstRaw_Nm]  "TCS_TrqReqst_Raw"
  [TrqRequst_Act_Nm] -> Saturation Dynamic2/2
  VehSpd_SlipTarget_mps/1 -> Add9/1
  Add9/1 -> Add1/1
  [Verr_mps] -> Relational Operator7/1
  Cal_DeltaV_mps/1 -> Relational Operator7/2
  Relational Operator7/1 -> Latch_on/1(Set), Logical Operator2/1  "TCS_Trigger"
  [TCS_TrqReqstRaw_Nm] -> Unit Delay4/1
  Logical Operator2/1 -> Logical Operator1/1
  Relational Operator8/1 -> Logical Operator1/2  "fSat_Actuators"
  Cal_DeltaV_mps1/1 -> Relational Operator8/2
  Logical Operator1/1 -> RisingTimer/1(Set)
  ResetDelay/1 -> RisingTimer/2(Timer)
  RisingTimer/1(TCSExit) -> Logical Operator3/1
  Logical Operator3/1 -> Latch_on/2(Reset)  "TCS_ExitFinal"
  Latch_on/1(flg_TCSActv) -> TCSR_flgActv/1, [TCS_Actv]
  [TCS_Actv] -> Switch6/2
  Verror_Reset/1 -> Switch6/3
  Switch6/1 -> Product/1, Add2/2  "Verror_mps"
  Product/1 -> [P_Portion], Add7/1  "P_out"
  [TCS_Actv] -> Detect Rise Positive/1
  [P_Portion] -> Unit Delay1/1
  Add4/1 -> Switch/1
  Unit Delay1/1 -> Add4/2
  [VehSpd_Ref_mps] -> Add5/1, VehicleStableTarget_mps/1
  VehicleStableTarget_mps/1 -> Add5/2
  Add5/1 -> Add10/2
  [VehSpd_RA_mps] -> Add10/1
  Add10/1 -> Relational Operator/1
  Verror/1 -> Relational Operator/2
  Relational Operator/1 -> Logical Operator4/1
  [TCS_Actv] -> Logical Operator4/2
  Logical Operator4/1 -> Switch1/2  "flg_I_FF"
  Trq_I_FF/1 -> Switch1/1
  Trq_IReset/1 -> Switch1/3
  Switch1/1 -> Add6/3  "Trq_I_FF"
  [P_Portion] -> Add11/2
  Add11/1 -> Saturation Dynamic/1
  [TCS_Actv] -> Switch2/2
  Switch7/1 -> Switch2/3
  [TrqRequst_Act_Nm] -> Switch7/1
  Verror1/1 -> Relational Operator1/2
  Add12/1 -> Relational Operator1/1
  [VehSpd_RA_mps] -> Add12/1
  Add13/1 -> Add12/2
  VehicleStableTarget_mps1/1 -> Add13/2
  [VehSpd_Ref_mps] -> VehicleStableTarget_mps1/1, Add13/1
  [TCS_TrqReqstRaw_Nm] -> Compare To Constant2/1, Relational Operator2/1
  [TrqRequst_Act_Nm] -> Relational Operator2/2
  Relational Operator1/1 -> Logical Operator5/1
  Relational Operator2/1 -> OR/1
  Logical Operator5/1 -> Unit Delay3/1, Switch7/2  "TCS_Inactive"
  Unit Delay3/1 -> [TCS_Inactive]
  [TCS_Inactive] -> Logical Operator3/2
  Unit Delay4/1 -> Relational Operator8/1
  VehSpdFL_mps/1 -> Saturation1/1  "VehSpdFL_mps"
  Saturation Dynamic1/1 -> Saturation Dynamic2/1
  TCS_TrqRequest_Max2/1 -> Saturation Dynamic1/1
  TCS_TrqRequest_Min2/1 -> Saturation Dynamic1/3
  Switch3/1 -> Add2/1
  Verror_Reset1/1 -> Switch3/1
  [Verr_Zore] -> Switch3/2
  Unit Delay5/1 -> Product2/2
  Product2/1 -> Compare To Constant/1
  Compare To Constant/1 -> [Verr_Zore]
  <StrWhlAng>/1 -> Abs/1
  Compare To Zero/1 -> Logical Operator6/1
  Abs/1 -> Compare To Constant1/1
  [VehSpd_RA_mps] -> Compare To Zero/1
  Compare To Constant1/1 -> Logical Operator6/2
  Unit Delay2/1 -> Switch7/3
  Switch5/1 -> TCSR_TrqRequestFinal_Nm/1
  Logical Operator6/1 -> Switch5/2
  [TrqRequst_Act_Nm] -> Switch5/3
  Compare To Constant2/1 -> OR/2
  OR/1 -> Logical Operator5/2

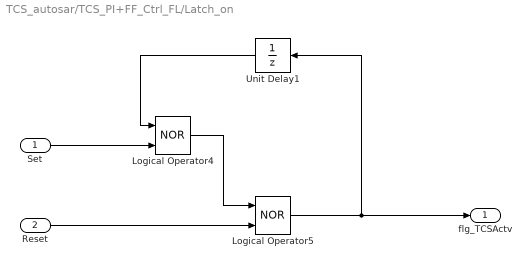
== system TCS_autosar/TCS_PI+FF_Ctrl_FL/Latch_on ==
  Set : Inport
  Reset : Inport  Port=2
  Logical Operator4 : Logic  Operator=NOR  AllPortsSameDT=off  OutDataTypeStr=boolean
  Logical Operator5 : Logic  Operator=NOR  AllPortsSameDT=off  OutDataTypeStr=boolean
  Unit Delay1 : UnitDelay  SampleTime=-1  HasFrameUpgradeWarning=on
  flg_TCSActv : Outport
  wires:
  Logical Operator5/1 -> flg_TCSActv/1, Unit Delay1/1
  Reset/1 -> Logical Operator5/2
  Unit Delay1/1 -> Logical Operator4/1
  Set/1 -> Logical Operator4/2
  Logical Operator4/1 -> Logical Operator5/1

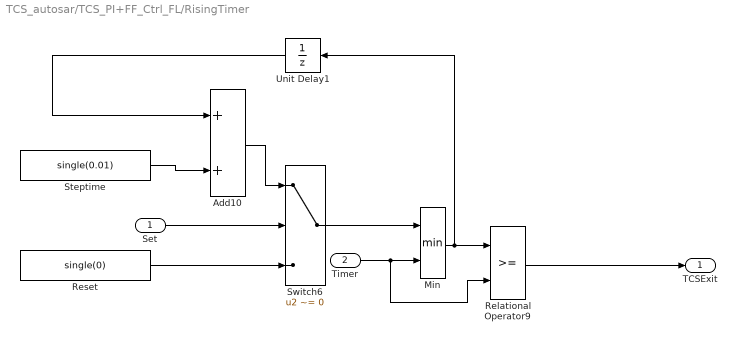
== system TCS_autosar/TCS_PI+FF_Ctrl_FL/RisingTimer ==
  Set : Inport
  Timer : Inport  Port=2
  Add10 : Sum
  Min : MinMax  Inputs=2
  Relational Operator9 : RelationalOperator  OutDataTypeStr=boolean  RndMeth=Simplest
  Reset : Constant  Value=single(0)
  Steptime : Constant  Value=single(0.01)
  Switch6 : Switch  Criteria=u2 ~= 0
  Unit Delay1 : UnitDelay  SampleTime=-1  HasFrameUpgradeWarning=on
  TCSExit : Outport
  wires:
  Add10/1 -> Switch6/1
  Set/1 -> Switch6/2
  Min/1 -> Unit Delay1/1, Relational Operator9/1
  Unit Delay1/1 -> Add10/1
  Timer/1 -> Relational Operator9/2, Min/2
  Reset/1 -> Switch6/3
  Relational Operator9/1 -> TCSExit/1
  Steptime/1 -> Add10/2
  Switch6/1 -> Min/1

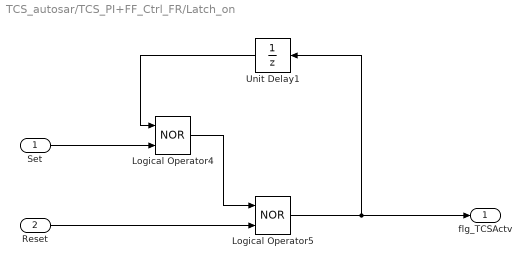
== system TCS_autosar/TCS_PI+FF_Ctrl_FR/Latch_on ==
  Set : Inport
  Reset : Inport  Port=2
  Logical Operator4 : Logic  Operator=NOR  AllPortsSameDT=off  OutDataTypeStr=boolean
  Logical Operator5 : Logic  Operator=NOR  AllPortsSameDT=off  OutDataTypeStr=boolean
  Unit Delay1 : UnitDelay  SampleTime=-1  HasFrameUpgradeWarning=on
  flg_TCSActv : Outport
  wires:
  Logical Operator4/1 -> Logical Operator5/1
  Set/1 -> Logical Operator4/2
  Unit Delay1/1 -> Logical Operator4/1
  Reset/1 -> Logical Operator5/2
  Logical Operator5/1 -> Unit Delay1/1, flg_TCSActv/1

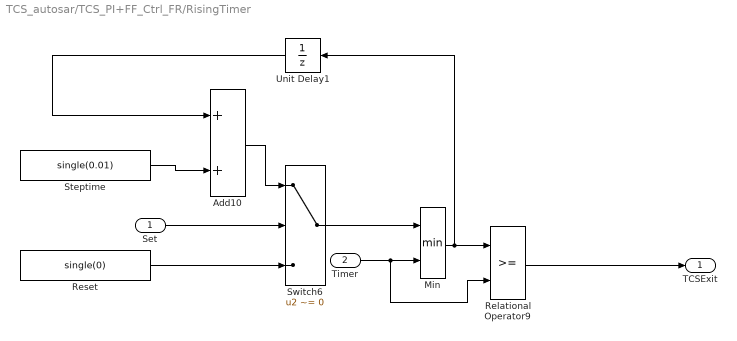
== system TCS_autosar/TCS_PI+FF_Ctrl_FR/RisingTimer ==
  Set : Inport
  Timer : Inport  Port=2
  Add10 : Sum
  Min : MinMax  Inputs=2
  Relational Operator9 : RelationalOperator  OutDataTypeStr=boolean  RndMeth=Simplest
  Reset : Constant  Value=single(0)
  Steptime : Constant  Value=single(0.01)
  Switch6 : Switch  Criteria=u2 ~= 0
  Unit Delay1 : UnitDelay  SampleTime=-1  HasFrameUpgradeWarning=on
  TCSExit : Outport
  wires:
  Switch6/1 -> Min/1
  Steptime/1 -> Add10/2
  Relational Operator9/1 -> TCSExit/1
  Reset/1 -> Switch6/3
  Timer/1 -> Min/2, Relational Operator9/2
  Unit Delay1/1 -> Add10/1
  Min/1 -> Relational Operator9/1, Unit Delay1/1
  Set/1 -> Switch6/2
  Add10/1 -> Switch6/1

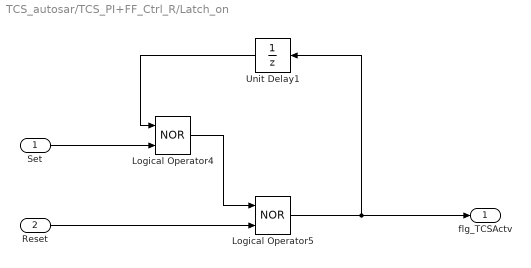
== system TCS_autosar/TCS_PI+FF_Ctrl_R/Latch_on ==
  Set : Inport
  Reset : Inport  Port=2
  Logical Operator4 : Logic  Operator=NOR  AllPortsSameDT=off  OutDataTypeStr=boolean
  Logical Operator5 : Logic  Operator=NOR  AllPortsSameDT=off  OutDataTypeStr=boolean
  Unit Delay1 : UnitDelay  SampleTime=-1  HasFrameUpgradeWarning=on
  flg_TCSActv : Outport
  wires:
  Logical Operator5/1 -> flg_TCSActv/1, Unit Delay1/1
  Reset/1 -> Logical Operator5/2
  Unit Delay1/1 -> Logical Operator4/1
  Set/1 -> Logical Operator4/2
  Logical Operator4/1 -> Logical Operator5/1

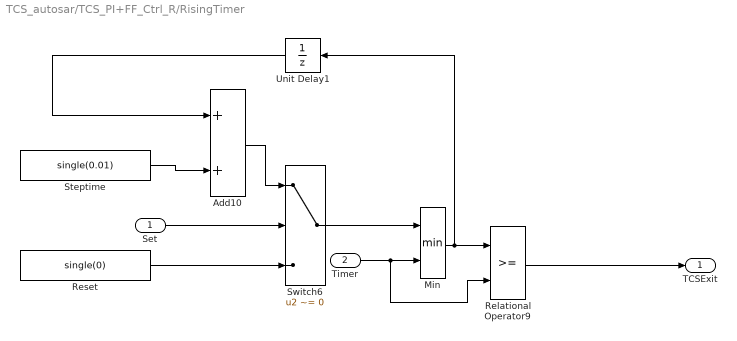
== system TCS_autosar/TCS_PI+FF_Ctrl_R/RisingTimer ==
  Set : Inport
  Timer : Inport  Port=2
  Add10 : Sum
  Min : MinMax  Inputs=2
  Relational Operator9 : RelationalOperator  OutDataTypeStr=boolean  RndMeth=Simplest
  Reset : Constant  Value=single(0)
  Steptime : Constant  Value=single(0.01)
  Switch6 : Switch  Criteria=u2 ~= 0
  Unit Delay1 : UnitDelay  SampleTime=-1  HasFrameUpgradeWarning=on
  TCSExit : Outport
  wires:
  Add10/1 -> Switch6/1
  Set/1 -> Switch6/2
  Min/1 -> Unit Delay1/1, Relational Operator9/1
  Unit Delay1/1 -> Add10/1
  Timer/1 -> Relational Operator9/2, Min/2
  Reset/1 -> Switch6/3
  Relational Operator9/1 -> TCSExit/1
  Steptime/1 -> Add10/2
  Switch6/1 -> Min/1
